simulink model "AME556_Project_Task3_v5"  (R2024b)
settings: Solver=daessc  StartTime=0.0  StopTime=10  FixedStep=0.0005  MaxStep=1e-3  RelTol=1e-2
InitFcn:
  | global params;
  | 
  | % Mass and geometry
  | params.m = 0.25;
  | params.l = 0.22;
  | params.mb = 8;
  | params.a = 0.25;
  | params.b = 0.15;
  | params.g = [0; 9.81; 0];
  | 
  | % Moment of inerita
  | Il_zz = params.m * params.l^2 / 12;
  | Ib_xx = params.mb * params.a^2 / 12;
  | Ib_yy = params.mb * params.b^2 / 12;
  | Ib_zz = params.mb * (params.a^2 + params.b^2) / 12;
  | params.Ib = diag([Ib_xx Ib_yy Ib_zz]);
  | 
  | % Spatial contact force parameters
  | Kp_g = 1e5;
  | Kd_g = 1e3;
  | 
  | % Ground contact positions
  | params.P1 = [0.0197; 0.0022; 0];
  | params.P2 = [0.1838; 0.0041; 0];
  | 
  | % State variables
  | q0 = [0.1; 0.45; 0; -pi/3; pi/2; -pi/6; pi/2]; % Initial states (before landing)
  | params.p_d = [0; 0.5; 0]; % Desired positions (after standing): [x_d; y_d; z_d];
  | params.theta_d = 0; % Desired angle
values from neighbouring files (symbols this model uses):
  dt = 0.04    [AME556_Project_Task3_Setup.m]
  N = 10    [AME556_Project_Task3_Setup.m]
undefined symbols (not defined in the file or in its folder): P1_world0, P2_world0, X, Y, Z
libraries: nesl_utility x27, sm_lib x23
settings Model: Creator=lewis  LastModifiedBy=zhaoshuai
settings SolverCC: DaesscMode=Balanced  AlgebraicLoopSolver=TrustRegion  MaxZcPerStep=1
settings DebuggingCC: UnconnectedInputMsg=warning  UnconnectedOutputMsg=warning  UnconnectedLineMsg=warning  SymbolicDimsDataTypeCodeGenerationDiagnostic=none
settings ModelReferenceCC: EnableRefExpFcnMdlSchedulingChecks=on
settings SFSimCC: CustomCodeUndefinedFunction=UseInterfaceOnly
settings RTWCC: GPUComputeCapability=3.5  DLArmComputeVersion=19.05
settings SimscapeCC: SimscapeLogType=all  SimscapeLogSimulationStatistics=on  SimscapeLogDataHistory=10000
settings ExplorerConfigSet: InternalSimMechanicsExplorerSettings="<ExplorerConfiguration><canonicalview>planar_xy</canonicalview><AnimationSetting><BasePlaybackSpeed>1.0</BasePlaybackSpeed><PlaybackSpeedFactor>1.0</PlaybackSpeedFactor></AnimationSetting><TilePanel><TileInfo><Tiles Columns=\"1\" Count=\"1\" Rows=\"1\"><Column Weight=\"1\"/><Row Weight=\"1\"/><Tile Height=\"1\" Width=\"1\" X=\"0\" Y=\"0\"/></Tiles></TileInfo><SceneInfo><SceneViewer><BGColor><R>0.60000002384185791</R><G>0.60000002384185791</G><B>0.60000002384185791</B></BGColor><Camera><DoPerspective>off</DoPerspective><Position><X>5.0000003994890756</X><Y>0.276248430591055971</Y><Z>5.31649358666460525</Z></Position><Center><X>5.0000003994890756</X><Y>0.276248430591055971</Y><Z>8.29291000314924531e-08</Z></Center><Up><X>0</X><Y>1</Y><Z>0</Z></Up><ViewLimDist>1</ViewLimDist><YLim>3.59969072164948445</YLim><XLim>5.40749999999999975</XLim></Camera></SceneViewer></SceneInfo></TilePanel><MechEditorPanel><Cameras/><GfxPanelCameraMap/><VideoCreator><PlaybackSpeedRatio>1.0</PlaybackSpeedRatio><FrameRate>60</FrameRate><VideoFormat>MPEG-4</VideoFormat><FrameSize>[1280 720]</FrameSize></VideoCreator></MechEditorPanel></ExplorerConfiguration>"

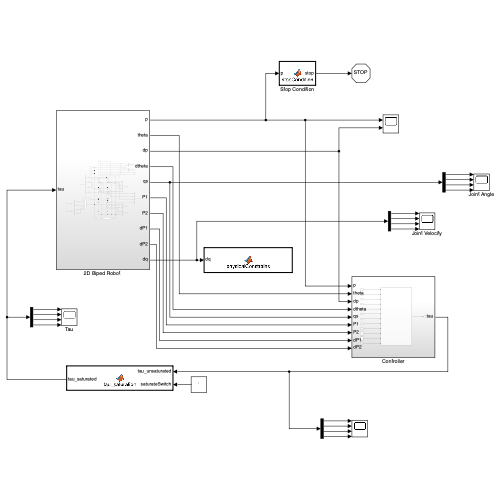
[thumbnail: Simulink's stored preview of the top-level diagram]
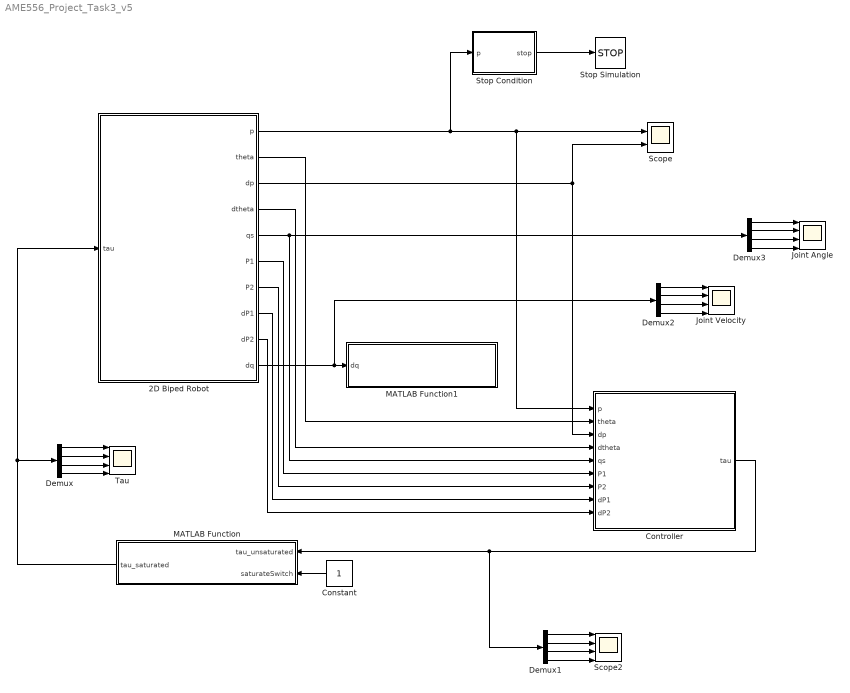
== system AME556_Project_Task3_v5 ==
  "2D Biped Robot " : Subsystem
  Constant : Constant
  Controller : Subsystem
  Demux{,1..3} (4 alike) : Demux
  Joint Angle : Scope  NumInputPorts=4
  Joint Velocity : Scope  NumInputPorts=4
  MATLAB Function : MATLAB Function  TreatAsAtomicUnit=on
  MATLAB Function1 : MATLAB Function  TreatAsAtomicUnit=on
  Scope : Scope  NumInputPorts=2
  Scope2 : Scope  NumInputPorts=4
  Stop Condition : MATLAB Function  TreatAsAtomicUnit=on
  Stop Simulation : Stop
  Tau : Scope  NumInputPorts=4
  wires:
  "2D Biped Robot "/1(p) -> Stop Condition/1(p), Scope/1, Controller/1(p)
  "2D Biped Robot "/2(theta) -> Controller/2(theta)
  "2D Biped Robot "/4(dtheta) -> Controller/4(dtheta)
  "2D Biped Robot "/6(P1) -> Controller/6(P1)
  "2D Biped Robot "/7(P2) -> Controller/7(P2)
  "2D Biped Robot "/8(dP1) -> Controller/8(dP1)
  "2D Biped Robot "/9(dP2) -> Controller/9(dP2)
  Stop Condition/1(stop) -> Stop Simulation/1
  "2D Biped Robot "/10(dq) -> Demux2/1, MATLAB Function1/1(dq)
  Constant/1 -> MATLAB Function/2(saturateSwitch)
  Demux/1 -> Tau/1
  Demux/2 -> Tau/2
  Demux/3 -> Tau/3
  Demux/4 -> Tau/4
  MATLAB Function/1(tau_saturated) -> Demux/1, "2D Biped Robot "/1(tau)
  Controller/1(tau) -> Demux1/1, MATLAB Function/1(tau_unsaturated)
  Demux1/1 -> Scope2/1
  Demux1/2 -> Scope2/2
  Demux1/3 -> Scope2/3
  Demux1/4 -> Scope2/4
  "2D Biped Robot "/3(dp) -> Scope/2, Controller/3(dp)
  Demux2/4 -> Joint Velocity/4
  Demux2/1 -> Joint Velocity/1
  Demux2/3 -> Joint Velocity/3
  Demux2/2 -> Joint Velocity/2
  Demux3/3 -> Joint Angle/3
  Demux3/1 -> Joint Angle/1
  Demux3/2 -> Joint Angle/2
  Demux3/4 -> Joint Angle/4
  "2D Biped Robot "/5(qs) -> Controller/5(qs), Demux3/1

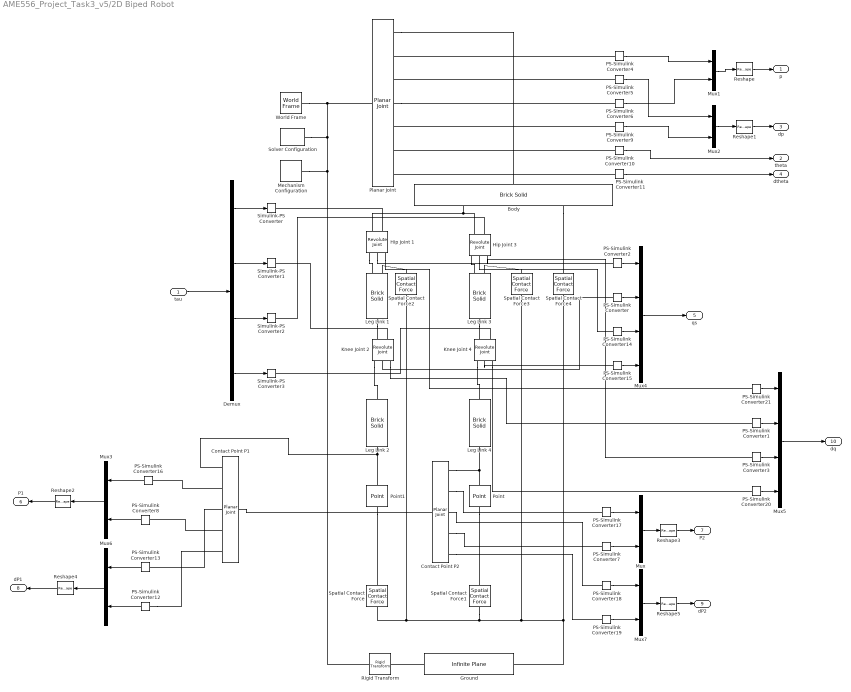
== system AME556_Project_Task3_v5/2D Biped Robot  ==
  tau : Inport
  Body : sm_lib/Body Elements/Brick Solid  BrickDimensions=[params.b params.a 0.1]  BrickDimensionsUnits=m  ExportEntireGeometry=on  InertiaType=Custom  BasedOnType=Density  Density=1000  DensityUnits=kg/m^3  Mass=params.mb  MassUnits=kg  CenterOfMass=[0 0 0]  CenterOfMassUnits=m  MomentsOfInertia=[0 0 Ib_zz]  MomentsOfInertiaUnits=kg*m^2  ProductsOfInertia=[0 0 0]  ProductsOfInertiaUnits=kg*m^2  GraphicType=FromGeometry  MarkerShape=Sphere  MarkerSize=10  GraphicVisPropType=SimpleVisualProperties  GraphicDiffuseColor=[0.5 0.5 0.5]  GraphicOpacity=1  GraphicSpecularColor=[0.5 0.5 0.5 1.0]  GraphicAmbientColor=[0.15 0.15 0.15 1.0]  GraphicEmissiveColor=[0.0 0.0 0.0 1.0]  GraphicShininess=75  DoExposeReferenceFrame=on  SerializedFrames=<Frames><Frame><Id>Frame1</Id><Value><Name>F</Name><Origin><Source>GeometricFeature</Source><FeatureName>-y surface</FeatureName></Origin><PrimaryAxis><DefinedDirection>+Z</DefinedDirection><Source>ReferenceFrame</Source><SourceDirection>+Z</SourceDirection><FeatureName></FeatureName></PrimaryAxis><SecondaryAxis><DefinedDirection>+X</DefinedDirection><Source>ReferenceFrame</Source><SourceDirection>+X</SourceDirection><FeatureName></FeatureName></SecondaryAxis></Value></Frame></Frames>
  Contact Point P1 : sm_lib/Joints/Planar Joint  JointMode=Normal  CompositeWrenchDir=FollowerOnBase  CompositeWrenchFrame=BaseFrame  SenseConstraintForce=off  SenseConstraintTorque=off  SenseTotalForce=off  SenseTotalTorque=off  PxPositionTargetSpecify=off  PxPositionTargetPriority=High  PxPositionTargetValue=P1_world0(1)  PxPositionTargetValueUnits=m  PxVelocityTargetSpecify=off  PxVelocityTargetPriority=High  PxVelocityTargetValue=0  PxVelocityTargetValueUnits=m/s  PxEquilibriumPosition=0  PxEquilibriumPositionUnits=m  PxSpringStiffness=0  PxSpringStiffnessUnits=N/m  PxDampingCoefficient=0  PxDampingCoefficientUnits=N/(m/s)  PxLowerLimitSpecify=off  PxLowerLimitBound=-1  PxLowerLimitBoundUnits=m  PxLowerLimitStiffness=1e6  PxLowerLimitStiffnessUnits=N/m  PxLowerLimitDamping=1e3  PxLowerLimitDampingUnits=N/(m/s)  PxLowerLimitTransitionRegionWidth=1e-4  PxLowerLimitTransitionRegionWidthUnits=m  PxUpperLimitSpecify=off  PxUpperLimitBound=1  PxUpperLimitBoundUnits=m  PxUpperLimitStiffness=1e6  PxUpperLimitStiffnessUnits=N/m  PxUpperLimitDamping=1e3  PxUpperLimitDampingUnits=N/(m/s)  PxUpperLimitTransitionRegionWidth=1e-4  PxUpperLimitTransitionRegionWidthUnits=m  PxTorqueActuationMode=NoTorque  PxMotionActuationMode=ComputedMotion  PxSensePosition=on  PxSenseVelocity=on  PxSenseAcceleration=off  PxSenseTorqueForce=off  PxSenseLowerLimitTorqueForce=off  PxSenseUpperLimitTorqueForce=off  PyPositionTargetSpecify=off  PyPositionTargetPriority=High  PyPositionTargetValue=P1_world0(2)  PyPositionTargetValueUnits=m  PyVelocityTargetSpecify=off  PyVelocityTargetPriority=High  PyVelocityTargetValue=0  PyVelocityTargetValueUnits=m/s  PyEquilibriumPosition=0  PyEquilibriumPositionUnits=m  PySpringStiffness=0  PySpringStiffnessUnits=N/m  PyDampingCoefficient=0  PyDampingCoefficientUnits=N/(m/s)  PyLowerLimitSpecify=off  PyLowerLimitBound=-1  PyLowerLimitBoundUnits=m  PyLowerLimitStiffness=1e6  PyLowerLimitStiffnessUnits=N/m  PyLowerLimitDamping=1e3  PyLowerLimitDampingUnits=N/(m/s)  PyLowerLimitTransitionRegionWidth=1e-4  PyLowerLimitTransitionRegionWidthUnits=m  PyUpperLimitSpecify=off  PyUpperLimitBound=1  PyUpperLimitBoundUnits=m  PyUpperLimitStiffness=1e6  PyUpperLimitStiffnessUnits=N/m  PyUpperLimitDamping=1e3  PyUpperLimitDampingUnits=N/(m/s)  PyUpperLimitTransitionRegionWidth=1e-4  PyUpperLimitTransitionRegionWidthUnits=m  PyTorqueActuationMode=NoTorque  PyMotionActuationMode=ComputedMotion  PySensePosition=on  PySenseVelocity=on  PySenseAcceleration=off  PySenseTorqueForce=off  PySenseLowerLimitTorqueForce=off  PySenseUpperLimitTorqueForce=off  RzPositionTargetSpecify=off  RzPositionTargetPriority=High  RzPositionTargetValue=q0(3)  RzPositionTargetValueUnits=deg  RzVelocityTargetSpecify=off  RzVelocityTargetPriority=High  RzVelocityTargetValue=0  RzVelocityTargetValueUnits=deg/s  RzEquilibriumPosition=0  RzEquilibriumPositionUnits=deg  RzSpringStiffness=0  RzSpringStiffnessUnits=N*m/deg  RzDampingCoefficient=0  RzDampingCoefficientUnits=N*m/(deg/s)  RzLowerLimitSpecify=off  RzLowerLimitBound=-90  RzLowerLimitBoundUnits=deg  RzLowerLimitStiffness=1e4  RzLowerLimitStiffnessUnits=N*m/deg  RzLowerLimitDamping=10  RzLowerLimitDampingUnits=N*m/(deg/s)  RzLowerLimitTransitionRegionWidth=0.1  RzLowerLimitTransitionRegionWidthUnits=deg  RzUpperLimitSpecify=off  RzUpperLimitBound=90  RzUpperLimitBoundUnits=deg  RzUpperLimitStiffness=1e4  RzUpperLimitStiffnessUnits=N*m/deg  RzUpperLimitDamping=10  RzUpperLimitDampingUnits=N*m/(deg/s)  RzUpperLimitTransitionRegionWidth=0.1  RzUpperLimitTransitionRegionWidthUnits=deg  RzTorqueActuationMode=NoTorque  RzMotionActuationMode=ComputedMotion  RzSensePosition=off  RzSenseVelocity=off  RzSenseAcceleration=off  RzSenseTorqueForce=off  RzSenseLowerLimitTorqueForce=off  RzSenseUpperLimitTorqueForce=off
  Contact Point P2 : sm_lib/Joints/Planar Joint  JointMode=Normal  CompositeWrenchDir=FollowerOnBase  CompositeWrenchFrame=BaseFrame  SenseConstraintForce=off  SenseConstraintTorque=off  SenseTotalForce=off  SenseTotalTorque=off  PxPositionTargetSpecify=off  PxPositionTargetPriority=High  PxPositionTargetValue=P2_world0(1)  PxPositionTargetValueUnits=m  PxVelocityTargetSpecify=off  PxVelocityTargetPriority=High  PxVelocityTargetValue=0  PxVelocityTargetValueUnits=m/s  PxEquilibriumPosition=0  PxEquilibriumPositionUnits=m  PxSpringStiffness=0  PxSpringStiffnessUnits=N/m  PxDampingCoefficient=0  PxDampingCoefficientUnits=N/(m/s)  PxLowerLimitSpecify=off  PxLowerLimitBound=-1  PxLowerLimitBoundUnits=m  PxLowerLimitStiffness=1e6  PxLowerLimitStiffnessUnits=N/m  PxLowerLimitDamping=1e3  PxLowerLimitDampingUnits=N/(m/s)  PxLowerLimitTransitionRegionWidth=1e-4  PxLowerLimitTransitionRegionWidthUnits=m  PxUpperLimitSpecify=off  PxUpperLimitBound=1  PxUpperLimitBoundUnits=m  PxUpperLimitStiffness=1e6  PxUpperLimitStiffnessUnits=N/m  PxUpperLimitDamping=1e3  PxUpperLimitDampingUnits=N/(m/s)  PxUpperLimitTransitionRegionWidth=1e-4  PxUpperLimitTransitionRegionWidthUnits=m  PxTorqueActuationMode=NoTorque  PxMotionActuationMode=ComputedMotion  PxSensePosition=on  PxSenseVelocity=on  PxSenseAcceleration=off  PxSenseTorqueForce=off  PxSenseLowerLimitTorqueForce=off  PxSenseUpperLimitTorqueForce=off  PyPositionTargetSpecify=off  PyPositionTargetPriority=High  PyPositionTargetValue=P2_world0(2)  PyPositionTargetValueUnits=m  PyVelocityTargetSpecify=off  PyVelocityTargetPriority=High  PyVelocityTargetValue=0  PyVelocityTargetValueUnits=m/s  PyEquilibriumPosition=0  PyEquilibriumPositionUnits=m  PySpringStiffness=0  PySpringStiffnessUnits=N/m  PyDampingCoefficient=0  PyDampingCoefficientUnits=N/(m/s)  PyLowerLimitSpecify=off  PyLowerLimitBound=-1  PyLowerLimitBoundUnits=m  PyLowerLimitStiffness=1e6  PyLowerLimitStiffnessUnits=N/m  PyLowerLimitDamping=1e3  PyLowerLimitDampingUnits=N/(m/s)  PyLowerLimitTransitionRegionWidth=1e-4  PyLowerLimitTransitionRegionWidthUnits=m  PyUpperLimitSpecify=off  PyUpperLimitBound=1  PyUpperLimitBoundUnits=m  PyUpperLimitStiffness=1e6  PyUpperLimitStiffnessUnits=N/m  PyUpperLimitDamping=1e3  PyUpperLimitDampingUnits=N/(m/s)  PyUpperLimitTransitionRegionWidth=1e-4  PyUpperLimitTransitionRegionWidthUnits=m  PyTorqueActuationMode=NoTorque  PyMotionActuationMode=ComputedMotion  PySensePosition=on  PySenseVelocity=on  PySenseAcceleration=off  PySenseTorqueForce=off  PySenseLowerLimitTorqueForce=off  PySenseUpperLimitTorqueForce=off  RzPositionTargetSpecify=off  RzPositionTargetPriority=High  RzPositionTargetValue=q0(3)  RzPositionTargetValueUnits=deg  RzVelocityTargetSpecify=off  RzVelocityTargetPriority=High  RzVelocityTargetValue=0  RzVelocityTargetValueUnits=deg/s  RzEquilibriumPosition=0  RzEquilibriumPositionUnits=deg  RzSpringStiffness=0  RzSpringStiffnessUnits=N*m/deg  RzDampingCoefficient=0  RzDampingCoefficientUnits=N*m/(deg/s)  RzLowerLimitSpecify=off  RzLowerLimitBound=-90  RzLowerLimitBoundUnits=deg  RzLowerLimitStiffness=1e4  RzLowerLimitStiffnessUnits=N*m/deg  RzLowerLimitDamping=10  RzLowerLimitDampingUnits=N*m/(deg/s)  RzLowerLimitTransitionRegionWidth=0.1  RzLowerLimitTransitionRegionWidthUnits=deg  RzUpperLimitSpecify=off  RzUpperLimitBound=90  RzUpperLimitBoundUnits=deg  RzUpperLimitStiffness=1e4  RzUpperLimitStiffnessUnits=N*m/deg  RzUpperLimitDamping=10  RzUpperLimitDampingUnits=N*m/(deg/s)  RzUpperLimitTransitionRegionWidth=0.1  RzUpperLimitTransitionRegionWidthUnits=deg  RzTorqueActuationMode=NoTorque  RzMotionActuationMode=ComputedMotion  RzSensePosition=off  RzSenseVelocity=off  RzSenseAcceleration=off  RzSenseTorqueForce=off  RzSenseLowerLimitTorqueForce=off  RzSenseUpperLimitTorqueForce=off
  Demux : Demux
  Ground : sm_lib/Curves and Surfaces/Infinite Plane  GraphicType=Rectangle  GraphicPlaneWidth=1  GraphicPlaneWidthUnits=m  GraphicPlaneHeight=10.5  GraphicPlaneHeightUnits=m  GraphicVisPropType=SimpleVisualProperties  GraphicDiffuseColor=[1 1 1]  GraphicOpacity=1  GraphicSpecularColor=[0.5 0.5 0.5 1.0]  GraphicAmbientColor=[0.15 0.15 0.15 1.0]  GraphicEmissiveColor=[0.0 0.0 0.0 1.0]  GraphicShininess=75
  Hip Joint 1 : sm_lib/Joints/Revolute Joint  JointMode=Normal  CompositeWrenchDir=FollowerOnBase  CompositeWrenchFrame=BaseFrame  SenseConstraintForce=off  SenseConstraintTorque=off  SenseTotalForce=off  SenseTotalTorque=off  PositionTargetSpecify=on  PositionTargetPriority=High  PositionTargetValue=params.q0(4)  PositionTargetValueUnits=rad  VelocityTargetSpecify=off  VelocityTargetPriority=High  VelocityTargetValue=0  VelocityTargetValueUnits=rad/s  EquilibriumPosition=0  EquilibriumPositionUnits=deg  SpringStiffness=0  SpringStiffnessUnits=N*m/deg  DampingCoefficient=0  DampingCoefficientUnits=N*m/(deg/s)  LowerLimitSpecify=on  LowerLimitBound=-120  LowerLimitBoundUnits=deg  LowerLimitStiffness=1e4  LowerLimitStiffnessUnits=N*m/deg  LowerLimitDamping=10  LowerLimitDampingUnits=N*m/(deg/s)  LowerLimitTransitionRegionWidth=0.1  LowerLimitTransitionRegionWidthUnits=deg  UpperLimitSpecify=on  UpperLimitBound=30  UpperLimitBoundUnits=deg  UpperLimitStiffness=1e4  UpperLimitStiffnessUnits=N*m/deg  UpperLimitDamping=10  UpperLimitDampingUnits=N*m/(deg/s)  UpperLimitTransitionRegionWidth=0.1  UpperLimitTransitionRegionWidthUnits=deg  TorqueActuationMode=InputTorque  MotionActuationMode=ComputedMotion  SensePosition=on  SenseVelocity=on  SenseAcceleration=off  SenseTorqueForce=off  SenseLowerLimitTorqueForce=off  SenseUpperLimitTorqueForce=off
  Hip Joint 3 : sm_lib/Joints/Revolute Joint  JointMode=Normal  CompositeWrenchDir=FollowerOnBase  CompositeWrenchFrame=BaseFrame  SenseConstraintForce=off  SenseConstraintTorque=off  SenseTotalForce=off  SenseTotalTorque=off  PositionTargetSpecify=on  PositionTargetPriority=High  PositionTargetValue=params.q0(6)  PositionTargetValueUnits=rad  VelocityTargetSpecify=off  VelocityTargetPriority=High  VelocityTargetValue=0  VelocityTargetValueUnits=rad/s  EquilibriumPosition=0  EquilibriumPositionUnits=deg  SpringStiffness=0  SpringStiffnessUnits=N*m/deg  DampingCoefficient=0  DampingCoefficientUnits=N*m/(deg/s)  LowerLimitSpecify=on  LowerLimitBound=-120  LowerLimitBoundUnits=deg  LowerLimitStiffness=1e4  LowerLimitStiffnessUnits=N*m/deg  LowerLimitDamping=10  LowerLimitDampingUnits=N*m/(deg/s)  LowerLimitTransitionRegionWidth=0.1  LowerLimitTransitionRegionWidthUnits=deg  UpperLimitSpecify=on  UpperLimitBound=30  UpperLimitBoundUnits=deg  UpperLimitStiffness=1e4  UpperLimitStiffnessUnits=N*m/deg  UpperLimitDamping=10  UpperLimitDampingUnits=N*m/(deg/s)  UpperLimitTransitionRegionWidth=0.1  UpperLimitTransitionRegionWidthUnits=deg  TorqueActuationMode=InputTorque  MotionActuationMode=ComputedMotion  SensePosition=on  SenseVelocity=on  SenseAcceleration=off  SenseTorqueForce=off  SenseLowerLimitTorqueForce=off  SenseUpperLimitTorqueForce=off
  Knee Joint 2 : sm_lib/Joints/Revolute Joint  JointMode=Normal  CompositeWrenchDir=FollowerOnBase  CompositeWrenchFrame=BaseFrame  SenseConstraintForce=off  SenseConstraintTorque=off  SenseTotalForce=off  SenseTotalTorque=off  PositionTargetSpecify=on  PositionTargetPriority=High  PositionTargetValue=params.q0(5)  PositionTargetValueUnits=rad  VelocityTargetSpecify=on  VelocityTargetPriority=High  VelocityTargetValue=0  VelocityTargetValueUnits=rad/s  EquilibriumPosition=0  EquilibriumPositionUnits=deg  SpringStiffness=0  SpringStiffnessUnits=N*m/deg  DampingCoefficient=0.035  DampingCoefficientUnits=N*m/(deg/s)  LowerLimitSpecify=on  LowerLimitBound=0  LowerLimitBoundUnits=deg  LowerLimitStiffness=1e4  LowerLimitStiffnessUnits=N*m/deg  LowerLimitDamping=10  LowerLimitDampingUnits=N*m/(deg/s)  LowerLimitTransitionRegionWidth=0.1  LowerLimitTransitionRegionWidthUnits=deg  UpperLimitSpecify=on  UpperLimitBound=160  UpperLimitBoundUnits=deg  UpperLimitStiffness=1e4  UpperLimitStiffnessUnits=N*m/deg  UpperLimitDamping=10  UpperLimitDampingUnits=N*m/(deg/s)  UpperLimitTransitionRegionWidth=0.1  UpperLimitTransitionRegionWidthUnits=deg  TorqueActuationMode=InputTorque  MotionActuationMode=ComputedMotion  SensePosition=on  SenseVelocity=on  SenseAcceleration=off  SenseTorqueForce=off  SenseLowerLimitTorqueForce=off  SenseUpperLimitTorqueForce=off
  Knee Joint 4 : sm_lib/Joints/Revolute Joint  JointMode=Normal  CompositeWrenchDir=FollowerOnBase  CompositeWrenchFrame=BaseFrame  SenseConstraintForce=off  SenseConstraintTorque=off  SenseTotalForce=off  SenseTotalTorque=off  PositionTargetSpecify=on  PositionTargetPriority=High  PositionTargetValue=params.q0(7)  PositionTargetValueUnits=rad  VelocityTargetSpecify=on  VelocityTargetPriority=High  VelocityTargetValue=0  VelocityTargetValueUnits=rad/s  EquilibriumPosition=0  EquilibriumPositionUnits=deg  SpringStiffness=0  SpringStiffnessUnits=N*m/deg  DampingCoefficient=0.035  DampingCoefficientUnits=N*m/(deg/s)  LowerLimitSpecify=on  LowerLimitBound=0  LowerLimitBoundUnits=deg  LowerLimitStiffness=1e4  LowerLimitStiffnessUnits=N*m/deg  LowerLimitDamping=10  LowerLimitDampingUnits=N*m/(deg/s)  LowerLimitTransitionRegionWidth=0.1  LowerLimitTransitionRegionWidthUnits=deg  UpperLimitSpecify=on  UpperLimitBound=160  UpperLimitBoundUnits=deg  UpperLimitStiffness=1e4  UpperLimitStiffnessUnits=N*m/deg  UpperLimitDamping=10  UpperLimitDampingUnits=N*m/(deg/s)  UpperLimitTransitionRegionWidth=0.1  UpperLimitTransitionRegionWidthUnits=deg  TorqueActuationMode=InputTorque  MotionActuationMode=ComputedMotion  SensePosition=on  SenseVelocity=on  SenseAcceleration=off  SenseTorqueForce=off  SenseLowerLimitTorqueForce=off  SenseUpperLimitTorqueForce=off
  Leg Link 1 : sm_lib/Body Elements/Brick Solid  BrickDimensions=[0.01 params.l 0.01]  BrickDimensionsUnits=m  ExportEntireGeometry=on  InertiaType=Custom  BasedOnType=Density  Density=1000  DensityUnits=kg/m^3  Mass=params.m  MassUnits=kg  CenterOfMass=[0 0 0]  CenterOfMassUnits=m  MomentsOfInertia=[0 0 Il_zz]  MomentsOfInertiaUnits=kg*m^2  ProductsOfInertia=[0 0 0]  ProductsOfInertiaUnits=kg*m^2  GraphicType=FromGeometry  MarkerShape=Sphere  MarkerSize=10  GraphicVisPropType=SimpleVisualProperties  GraphicDiffuseColor=[0.07451 0.6235 1]  GraphicOpacity=1  GraphicSpecularColor=[0.5 0.5 0.5 1.0]  GraphicAmbientColor=[0.15 0.15 0.15 1.0]  GraphicEmissiveColor=[0.0 0.0 0.0 1.0]  GraphicShininess=75  DoExposeReferenceFrame=off  SerializedFrames=<Frames><Frame><Id>Frame1</Id><Value><Name>top</Name><Origin><Source>GeometricFeature</Source><FeatureName>+y surface</FeatureName></Origin><PrimaryAxis><DefinedDirection>+Z</DefinedDirection><Source>ReferenceFrame</Source><SourceDirection>+Z</SourceDirection><FeatureName></FeatureName></PrimaryAxis><SecondaryAxis><DefinedDirection>+X</DefinedDirection><Source>ReferenceFrame</Source><SourceDirection>+X</SourceDirection><FeatureName></FeatureName></SecondaryAxis></Value></Frame><Frame><Id>Frame2</Id><Value><Name>bottom</Name><Origin><Source>GeometricFeature</Source><FeatureName>-y surface</FeatureName></Origin><PrimaryAxis><DefinedDirection>+Z</DefinedDirection><Source>ReferenceFrame</Source><SourceDirection>+Z</SourceDirection><FeatureName></FeatureName></PrimaryAxis><SecondaryAxis><DefinedDirection>+X</DefinedDirection><Source>ReferenceFrame</Source><SourceDirection>+X</SourceDirection><FeatureName></FeatureName></SecondaryAxis></Value></Frame></Frames>
  Leg Link 2 : sm_lib/Body Elements/Brick Solid  BrickDimensions=[0.01 params.l 0.01]  BrickDimensionsUnits=m  ExportEntireGeometry=off  InertiaType=Custom  BasedOnType=Density  Density=1000  DensityUnits=kg/m^3  Mass=params.m  MassUnits=kg  CenterOfMass=[0 0 0]  CenterOfMassUnits=m  MomentsOfInertia=[0 0 Il_zz]  MomentsOfInertiaUnits=kg*m^2  ProductsOfInertia=[0 0 0]  ProductsOfInertiaUnits=kg*m^2  GraphicType=FromGeometry  MarkerShape=Sphere  MarkerSize=10  GraphicVisPropType=SimpleVisualProperties  GraphicDiffuseColor=[1 0 0]  GraphicOpacity=1  GraphicSpecularColor=[0.5 0.5 0.5 1.0]  GraphicAmbientColor=[0.15 0.15 0.15 1.0]  GraphicEmissiveColor=[0.0 0.0 0.0 1.0]  GraphicShininess=75  DoExposeReferenceFrame=off  SerializedFrames=<Frames><Frame><Id>Frame1</Id><Value><Name>top</Name><Origin><Source>GeometricFeature</Source><FeatureName>+y surface</FeatureName></Origin><PrimaryAxis><DefinedDirection>+Z</DefinedDirection><Source>ReferenceFrame</Source><SourceDirection>+Z</SourceDirection><FeatureName></FeatureName></PrimaryAxis><SecondaryAxis><DefinedDirection>+X</DefinedDirection><Source>ReferenceFrame</Source><SourceDirection>+X</SourceDirection><FeatureName></FeatureName></SecondaryAxis></Value></Frame><Frame><Id>Frame2</Id><Value><Name>bottom</Name><Origin><Source>GeometricFeature</Source><FeatureName>-y surface</FeatureName></Origin><PrimaryAxis><DefinedDirection>+Z</DefinedDirection><Source>ReferenceFrame</Source><SourceDirection>+Z</SourceDirection><FeatureName></FeatureName></PrimaryAxis><SecondaryAxis><DefinedDirection>+X</DefinedDirection><Source>ReferenceFrame</Source><SourceDirection>+X</SourceDirection><FeatureName></FeatureName></SecondaryAxis></Value></Frame></Frames>
  Leg Link 3 : sm_lib/Body Elements/Brick Solid  BrickDimensions=[0.01 params.l 0.01]  BrickDimensionsUnits=m  ExportEntireGeometry=on  InertiaType=Custom  BasedOnType=Density  Density=1000  DensityUnits=kg/m^3  Mass=params.m  MassUnits=kg  CenterOfMass=[0 0 0]  CenterOfMassUnits=m  MomentsOfInertia=[0 0 Il_zz]  MomentsOfInertiaUnits=kg*m^2  ProductsOfInertia=[0 0 0]  ProductsOfInertiaUnits=kg*m^2  GraphicType=FromGeometry  MarkerShape=Sphere  MarkerSize=10  GraphicVisPropType=SimpleVisualProperties  GraphicDiffuseColor=[0 1 0]  GraphicOpacity=1  GraphicSpecularColor=[0.5 0.5 0.5 1.0]  GraphicAmbientColor=[0.15 0.15 0.15 1.0]  GraphicEmissiveColor=[0.0 0.0 0.0 1.0]  GraphicShininess=75  DoExposeReferenceFrame=off  SerializedFrames=<Frames><Frame><Id>Frame1</Id><Value><Name>top</Name><Origin><Source>GeometricFeature</Source><FeatureName>+y surface</FeatureName></Origin><PrimaryAxis><DefinedDirection>+Z</DefinedDirection><Source>ReferenceFrame</Source><SourceDirection>+Z</SourceDirection><FeatureName></FeatureName></PrimaryAxis><SecondaryAxis><DefinedDirection>+X</DefinedDirection><Source>ReferenceFrame</Source><SourceDirection>+X</SourceDirection><FeatureName></FeatureName></SecondaryAxis></Value></Frame><Frame><Id>Frame2</Id><Value><Name>bottom</Name><Origin><Source>GeometricFeature</Source><FeatureName>-y surface</FeatureName></Origin><PrimaryAxis><DefinedDirection>+Z</DefinedDirection><Source>ReferenceFrame</Source><SourceDirection>+Z</SourceDirection><FeatureName></FeatureName></PrimaryAxis><SecondaryAxis><DefinedDirection>+X</DefinedDirection><Source>ReferenceFrame</Source><SourceDirection>+X</SourceDirection><FeatureName></FeatureName></SecondaryAxis></Value></Frame></Frames>
  Leg Link 4 : sm_lib/Body Elements/Brick Solid  BrickDimensions=[0.01 params.l 0.01]  BrickDimensionsUnits=m  ExportEntireGeometry=off  InertiaType=Custom  BasedOnType=Density  Density=1000  DensityUnits=kg/m^3  Mass=params.m  MassUnits=kg  CenterOfMass=[0 0 0]  CenterOfMassUnits=m  MomentsOfInertia=[0 0 Il_zz]  MomentsOfInertiaUnits=kg*m^2  ProductsOfInertia=[0 0 0]  ProductsOfInertiaUnits=kg*m^2  GraphicType=FromGeometry  MarkerShape=Sphere  MarkerSize=10  GraphicVisPropType=SimpleVisualProperties  GraphicDiffuseColor=[1 1 0]  GraphicOpacity=1  GraphicSpecularColor=[0.5 0.5 0.5 1.0]  GraphicAmbientColor=[0.15 0.15 0.15 1.0]  GraphicEmissiveColor=[0.0 0.0 0.0 1.0]  GraphicShininess=75  DoExposeReferenceFrame=off  SerializedFrames=<Frames><Frame><Id>Frame1</Id><Value><Name>top</Name><Origin><Source>GeometricFeature</Source><FeatureName>+y surface</FeatureName></Origin><PrimaryAxis><DefinedDirection>+Z</DefinedDirection><Source>ReferenceFrame</Source><SourceDirection>+Z</SourceDirection><FeatureName></FeatureName></PrimaryAxis><SecondaryAxis><DefinedDirection>+X</DefinedDirection><Source>ReferenceFrame</Source><SourceDirection>+X</SourceDirection><FeatureName></FeatureName></SecondaryAxis></Value></Frame><Frame><Id>Frame2</Id><Value><Name>bottom</Name><Origin><Source>GeometricFeature</Source><FeatureName>-y surface</FeatureName></Origin><PrimaryAxis><DefinedDirection>+Z</DefinedDirection><Source>ReferenceFrame</Source><SourceDirection>+Z</SourceDirection><FeatureName></FeatureName></PrimaryAxis><SecondaryAxis><DefinedDirection>+X</DefinedDirection><Source>ReferenceFrame</Source><SourceDirection>+X</SourceDirection><FeatureName></FeatureName></SecondaryAxis></Value></Frame></Frames>
  Mechanism Configuration : sm_lib/Utilities/Mechanism Configuration  UniformGravity=Constant  GravityVector=-params.g  GravityVectorUnits=m/s^2  LinearizationDelta=0.001  JointModeTransitionNonlinearIterations=2
  Mux{,1..3,6..7} (6 alike) : Mux  Inputs=2
  Mux4 : Mux
  Mux5 : Mux
  PS-Simulink Converter{,1..21} (22 alike) : nesl_utility/PS-Simulink Converter  PhysicalDomain=network_engine_domain  SubClassName=ps_output  LeftPortType=input  RightPortType=output  PseudoPeriodic=off  Frequencies=[]  VectorFormat=inherit  Unit=inherit  AffineConversion=off
  Planar Joint : sm_lib/Joints/Planar Joint  JointMode=Normal  CompositeWrenchDir=FollowerOnBase  CompositeWrenchFrame=BaseFrame  SenseConstraintForce=off  SenseConstraintTorque=off  SenseTotalForce=off  SenseTotalTorque=off  PxPositionTargetSpecify=on  PxPositionTargetPriority=High  PxPositionTargetValue=params.q0(1)  PxPositionTargetValueUnits=m  PxVelocityTargetSpecify=off  PxVelocityTargetPriority=High  PxVelocityTargetValue=0  PxVelocityTargetValueUnits=m/s  PxEquilibriumPosition=0  PxEquilibriumPositionUnits=m  PxSpringStiffness=0  PxSpringStiffnessUnits=N/m  PxDampingCoefficient=0  PxDampingCoefficientUnits=N/(m/s)  PxLowerLimitSpecify=off  PxLowerLimitBound=-1  PxLowerLimitBoundUnits=m  PxLowerLimitStiffness=1e6  PxLowerLimitStiffnessUnits=N/m  PxLowerLimitDamping=1e3  PxLowerLimitDampingUnits=N/(m/s)  PxLowerLimitTransitionRegionWidth=1e-4  PxLowerLimitTransitionRegionWidthUnits=m  PxUpperLimitSpecify=off  PxUpperLimitBound=1  PxUpperLimitBoundUnits=m  PxUpperLimitStiffness=1e6  PxUpperLimitStiffnessUnits=N/m  PxUpperLimitDamping=1e3  PxUpperLimitDampingUnits=N/(m/s)  PxUpperLimitTransitionRegionWidth=1e-4  PxUpperLimitTransitionRegionWidthUnits=m  PxTorqueActuationMode=NoTorque  PxMotionActuationMode=ComputedMotion  PxSensePosition=on  PxSenseVelocity=on  PxSenseAcceleration=off  PxSenseTorqueForce=off  PxSenseLowerLimitTorqueForce=off  PxSenseUpperLimitTorqueForce=off  PyPositionTargetSpecify=on  PyPositionTargetPriority=High  PyPositionTargetValue=params.q0(2)  PyPositionTargetValueUnits=m  PyVelocityTargetSpecify=off  PyVelocityTargetPriority=High  PyVelocityTargetValue=0  PyVelocityTargetValueUnits=m/s  PyEquilibriumPosition=0  PyEquilibriumPositionUnits=m  PySpringStiffness=0  PySpringStiffnessUnits=N/m  PyDampingCoefficient=0  PyDampingCoefficientUnits=N/(m/s)  PyLowerLimitSpecify=off  PyLowerLimitBound=-1  PyLowerLimitBoundUnits=m  PyLowerLimitStiffness=1e6  PyLowerLimitStiffnessUnits=N/m  PyLowerLimitDamping=1e3  PyLowerLimitDampingUnits=N/(m/s)  PyLowerLimitTransitionRegionWidth=1e-4  PyLowerLimitTransitionRegionWidthUnits=m  PyUpperLimitSpecify=off  PyUpperLimitBound=1  PyUpperLimitBoundUnits=m  PyUpperLimitStiffness=1e6  PyUpperLimitStiffnessUnits=N/m  PyUpperLimitDamping=1e3  PyUpperLimitDampingUnits=N/(m/s)  PyUpperLimitTransitionRegionWidth=1e-4  PyUpperLimitTransitionRegionWidthUnits=m  PyTorqueActuationMode=NoTorque  PyMotionActuationMode=ComputedMotion  PySensePosition=on  PySenseVelocity=on  PySenseAcceleration=off  PySenseTorqueForce=off  PySenseLowerLimitTorqueForce=off  PySenseUpperLimitTorqueForce=off  RzPositionTargetSpecify=on  RzPositionTargetPriority=High  RzPositionTargetValue=params.q0(3)  RzPositionTargetValueUnits=rad  RzVelocityTargetSpecify=off  RzVelocityTargetPriority=High  RzVelocityTargetValue=0  RzVelocityTargetValueUnits=deg/s  RzEquilibriumPosition=0  RzEquilibriumPositionUnits=deg  RzSpringStiffness=0  RzSpringStiffnessUnits=N*m/deg  RzDampingCoefficient=0  RzDampingCoefficientUnits=N*m/(deg/s)  RzLowerLimitSpecify=off  RzLowerLimitBound=-90  RzLowerLimitBoundUnits=deg  RzLowerLimitStiffness=1e4  RzLowerLimitStiffnessUnits=N*m/deg  RzLowerLimitDamping=10  RzLowerLimitDampingUnits=N*m/(deg/s)  RzLowerLimitTransitionRegionWidth=0.1  RzLowerLimitTransitionRegionWidthUnits=deg  RzUpperLimitSpecify=off  RzUpperLimitBound=90  RzUpperLimitBoundUnits=deg  RzUpperLimitStiffness=1e4  RzUpperLimitStiffnessUnits=N*m/deg  RzUpperLimitDamping=10  RzUpperLimitDampingUnits=N*m/(deg/s)  RzUpperLimitTransitionRegionWidth=0.1  RzUpperLimitTransitionRegionWidthUnits=deg  RzTorqueActuationMode=NoTorque  RzMotionActuationMode=ComputedMotion  RzSensePosition=on  RzSenseVelocity=on  RzSenseAcceleration=off  RzSenseTorqueForce=off  RzSenseLowerLimitTorqueForce=off  RzSenseUpperLimitTorqueForce=off
  Point : sm_lib/Curves and Surfaces/Point  GraphicType=Marker  MarkerShape=Sphere  MarkerSize=10  GraphicVisPropType=SimpleVisualProperties  GraphicDiffuseColor=[1 1 0.06667]  GraphicOpacity=1  GraphicSpecularColor=[0.5 0.5 0.5 1.0]  GraphicAmbientColor=[0.15 0.15 0.15 1.0]  GraphicEmissiveColor=[0.0 0.0 0.0 1.0]  GraphicShininess=75
  Point1 : sm_lib/Curves and Surfaces/Point  GraphicType=Marker  MarkerShape=Sphere  MarkerSize=10  GraphicVisPropType=SimpleVisualProperties  GraphicDiffuseColor=[1 0 0]  GraphicOpacity=1  GraphicSpecularColor=[0.5 0.5 0.5 1.0]  GraphicAmbientColor=[0.15 0.15 0.15 1.0]  GraphicEmissiveColor=[0.0 0.0 0.0 1.0]  GraphicShininess=75
  Reshape{,1..5} (6 alike) : Reshape  OutputDimensionality=Customize  OutputDimensions=[2,1]
  Rigid Transform : sm_lib/Frames and Transforms/Rigid Transform  RotationMethod=AlignedAxes  FollAlignAxisA=+X  BaseAlignAxisA=+Z  FollAlignAxisB=+Y  BaseAlignAxisB=+X  RotationStandardAxis=+Z  RotationAngle=0  RotationAngleUnits=deg  RotationArbitraryAxis=[0 0 1]  RotationSequenceAxes=FollowerAxes  RotationSequence=XYX  RotationSequenceAngles=[0 0 0]  RotationSequenceAnglesUnits=deg  RotationMatrix=[1 0 0;0 1 0;0 0 1]  Quaternion=[1 0 0 0]  TranslationMethod=StandardAxis  TranslationCartesianOffset=[0 0 0]  TranslationCartesianOffsetUnits=m  TranslationStandardAxis=+X  TranslationStandardOffset=5  TranslationStandardOffsetUnits=m  TranslationROffset=0  TranslationROffsetUnits=m  TranslationThetaOffset=0  TranslationThetaOffsetUnits=deg  TranslationZOffset=0  TranslationZOffsetUnits=m
  Simulink-PS Converter{,1..3} (4 alike) : nesl_utility/Simulink-PS Converter  PhysicalDomain=network_engine_domain  SubClassName=ps_input  LeftPortType=input  RightPortType=output  PseudoPeriodic=off  Frequencies=[]  NoiseDistribution=none  NoiseParameters=[]  Unit=1  AffineConversion=off  FilteringAndDerivatives=provide  SimscapeFilterOrder=1  InputFilterTimeConstant=0.001  UdotUserProvided=0
  Solver Configuration : nesl_utility/Solver Configuration  PhysicalDomain=network_engine_domain  SubClassName=solver  LeftPortType=input  RightPortType=generic  Tones=[]  Harmonics=[]  SimulateNoise=off  Profile=off  UseLocalSampling=off  EnableSwitchedLinearOptims=on  FrequencyDomain=off  UseCCode=off  RelTol=0.001  AbsTol=1e-06  MinStep=1e-09  ToWorkspace=off  RevertToSquareIcSolve=off  NumHomotopyIterations=100  PhasorMode=off  PhasorModeNumHarmonics=1  ConsistencySolver=NEWTON_XTOL_AFTER_FTOL  IndexReductionMethod=DerivativeReplacement  DoDC=off  ResidualTolerance=1e-09  ConsistencyTolSource=GLOBAL  ConsistencyAbsTol=0.001  ConsistencyRelTol=0.001  ConsistencyTolFactor=0.001  UseLocalSolver=off  LocalSolverChoice=NE_BACKWARD_EULER_ADVANCER  ResolveIndetEquations=on  FunctionEvalNumThread=1  LocalSolverSampleTime=0.001  DoFixedCost=off  MaxNonlinIter=3  MaxModeIter=2  ComputeImpulses=off  ImpulseIterations=2  LinearAlgebra=auto  LinearAlgebraNumThread=0  EquationFormulation=NE_TIME_EF  DelaysMemoryBudget=1024  AutomaticFiltering=on  FilteringTimeConstant=0.001  PartitionStorageMethod=AS_NEEDED  PartitionMemoryBudget=1024  PartitionMethod=ROBUST  MultibodyUseLocalSolver=off  MultibodyLocalSolverChoice=ODE1  MultibodyLocalSolverSampleTime=0.001
  Spatial Contact Force{,1..4} (5 alike) : sm_lib/Forces and Torques/Spatial Contact Force  NormalForceType=SmoothSpringDamper  NormalStiffness=Kp_g  NormalStiffnessUnits=N/m  NormalDamping=Kd_g  NormalDampingUnits=N/(m/s)  NormalTransitionRegionWidth=1e-4  NormalTransitionRegionWidthUnits=m  FrictionType=SmoothStickSlip  CoefficientOfStaticFriction=Cof_s  CoefficientOfDynamicFriction=Cof_d  FrictionalCriticalVelocity=1e-3  FrictionalCriticalVelocityUnits=m/s  SenseContactSignal=off  SensePenetrationDepth=off  SenseSeparationDistance=off  SenseNormalForceMagnitude=off  SenseFrictionalForceMagnitude=off  SenseNormalVelocity=off  SenseTangentialVelocity=off  SenseContactBaseRotation=off  SenseContactBaseTranslation=off  SenseContactFollowerRotation=off  SenseContactFollowerTranslation=off  ZeroCrossDetectContactStartAndEnd=off
  World Frame : sm_lib/Frames and Transforms/World Frame
  p : Outport
  theta : Outport  Port=2
  dp : Outport  Port=3
  dtheta : Outport  Port=4
  qs : Outport  Port=5
  P1 : Outport  Port=6
  P2 : Outport  Port=7
  dP1 : Outport  Port=8
  dP2 : Outport  Port=9
  dq : Outport  Port=10
  wires:
  PS-Simulink Converter4/1 -> Mux1/1
  PS-Simulink Converter6/1 -> Mux1/2
  PS-Simulink Converter5/1 -> Mux2/1
  Demux/1 -> Simulink-PS Converter/1
  Demux/2 -> Simulink-PS Converter1/1
  Demux/3 -> Simulink-PS Converter2/1
  PS-Simulink Converter8/1 -> Mux3/2
  PS-Simulink Converter9/1 -> Mux2/2
  PS-Simulink Converter11/1 -> dtheta/1
  PS-Simulink Converter10/1 -> theta/1
  PS-Simulink Converter16/1 -> Mux3/1
  PS-Simulink Converter17/1 -> Mux/1
  PS-Simulink Converter7/1 -> Mux/2
  Mux/1 -> Reshape3/1
  Mux1/1 -> Reshape/1
  Mux2/1 -> Reshape1/1
  Mux3/1 -> Reshape2/1
  Reshape/1 -> p/1
  Reshape1/1 -> dp/1
  Reshape3/1 -> P2/1
  Reshape2/1 -> P1/1
  PS-Simulink Converter15/1 -> Mux4/4
  PS-Simulink Converter14/1 -> Mux4/3
  PS-Simulink Converter/1 -> Mux4/2
  PS-Simulink Converter2/1 -> Mux4/1
  Mux4/1 -> qs/1
  Demux/4 -> Simulink-PS Converter3/1
  tau/1 -> Demux/1
  Mux6/1 -> Reshape4/1
  Reshape4/1 -> dP1/1
  PS-Simulink Converter13/1 -> Mux6/1
  PS-Simulink Converter12/1 -> Mux6/2
  PS-Simulink Converter18/1 -> Mux7/1
  Mux7/1 -> Reshape5/1
  Reshape5/1 -> dP2/1
  PS-Simulink Converter19/1 -> Mux7/2
  Mux5/1 -> dq/1
  PS-Simulink Converter1/1 -> Mux5/2
  PS-Simulink Converter3/1 -> Mux5/3
  PS-Simulink Converter21/1 -> Mux5/1
  PS-Simulink Converter20/1 -> Mux5/4
  connections:
  Spatial Contact Force4/LConn1 -- Spatial Contact Force2/LConn1 -- Spatial Contact Force/LConn1 -- Spatial Contact Force1/LConn1 -- Spatial Contact Force3/LConn1 -- Ground/RConn1
  Hip Joint 1/LConn1 -- Hip Joint 3/LConn1 -- Body/LConn1
  Planar Joint/RConn1 -- Body/RConn1
  Hip Joint 1/RConn1 -- Leg Link 1/LConn1
  Hip Joint 3/RConn1 -- Leg Link 3/LConn1
  Leg Link 1/RConn1 -- Knee Joint 2/LConn1
  Knee Joint 2/RConn1 -- Leg Link 2/LConn1
  Knee Joint 4/RConn1 -- Leg Link 4/LConn1
  Leg Link 3/RConn1 -- Knee Joint 4/LConn1
  Leg Link 1/LConn2 -- Spatial Contact Force2/RConn1
  Leg Link 3/LConn2 -- Spatial Contact Force3/RConn1
  Body/LConn2 -- Spatial Contact Force4/RConn1
  PS-Simulink Converter/LConn1 -- Knee Joint 2/RConn2
  Hip Joint 1/RConn2 -- PS-Simulink Converter2/LConn1
  PS-Simulink Converter4/LConn1 -- Planar Joint/RConn2
  PS-Simulink Converter5/LConn1 -- Planar Joint/RConn3
  Planar Joint/RConn4 -- PS-Simulink Converter6/LConn1
  Point1/RConn1 -- Spatial Contact Force/RConn1
  Point/RConn1 -- Spatial Contact Force1/RConn1
  Contact Point P2/RConn1 -- Point/LConn1 -- Leg Link 4/RConn1
  Contact Point P1/RConn1 -- Point1/LConn1 -- Leg Link 2/RConn1
  PS-Simulink Converter9/LConn1 -- Planar Joint/RConn5
  PS-Simulink Converter10/LConn1 -- Planar Joint/RConn6
  PS-Simulink Converter11/LConn1 -- Planar Joint/RConn7
  Hip Joint 3/RConn2 -- PS-Simulink Converter14/LConn1
  Knee Joint 4/RConn2 -- PS-Simulink Converter15/LConn1
  Hip Joint 1/LConn2 -- Simulink-PS Converter/RConn1
  Knee Joint 2/LConn2 -- Simulink-PS Converter1/RConn1
  Hip Joint 3/LConn2 -- Simulink-PS Converter2/RConn1
  Knee Joint 4/LConn2 -- Simulink-PS Converter3/RConn1
  Contact Point P1/RConn2 -- PS-Simulink Converter16/LConn1
  Contact Point P2/RConn2 -- PS-Simulink Converter17/LConn1
  World Frame/RConn1 -- Solver Configuration/RConn1 -- Contact Point P1/LConn1 -- Rigid Transform/LConn1 -- Contact Point P2/LConn1 -- Mechanism Configuration/RConn1 -- Planar Joint/LConn1
  Ground/LConn1 -- Rigid Transform/RConn1
  Contact Point P1/RConn4 -- PS-Simulink Converter8/LConn1
  Contact Point P1/RConn3 -- PS-Simulink Converter13/LConn1
  PS-Simulink Converter12/LConn1 -- Contact Point P1/RConn5
  Contact Point P2/RConn4 -- PS-Simulink Converter7/LConn1
  Contact Point P2/RConn3 -- PS-Simulink Converter18/LConn1
  Contact Point P2/RConn5 -- PS-Simulink Converter19/LConn1
  Hip Joint 1/RConn3 -- PS-Simulink Converter21/LConn1
  Knee Joint 2/RConn3 -- PS-Simulink Converter1/LConn1
  Hip Joint 3/RConn3 -- PS-Simulink Converter3/LConn1
  Knee Joint 4/RConn3 -- PS-Simulink Converter20/LConn1

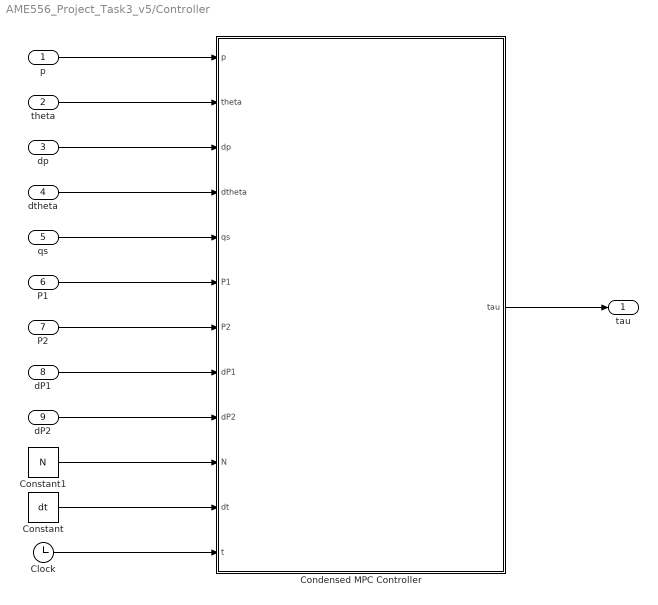
== system AME556_Project_Task3_v5/Controller ==
  p : Inport
  theta : Inport  Port=2
  dp : Inport  Port=3
  dtheta : Inport  Port=4
  qs : Inport  Port=5
  P1 : Inport  Port=6
  P2 : Inport  Port=7
  dP1 : Inport  Port=8
  dP2 : Inport  Port=9
  Clock : Clock
  Condensed MPC Controller : MATLAB Function  TreatAsAtomicUnit=on
  Constant : Constant  Value=dt
  Constant1 : Constant  Value=N
  tau : Outport
  wires:
  Condensed MPC Controller/1(tau) -> tau/1
  p/1 -> Condensed MPC Controller/1(p)
  theta/1 -> Condensed MPC Controller/2(theta)
  dp/1 -> Condensed MPC Controller/3(dp)
  P1/1 -> Condensed MPC Controller/6(P1)
  P2/1 -> Condensed MPC Controller/7(P2)
  dP1/1 -> Condensed MPC Controller/8(dP1)
  dP2/1 -> Condensed MPC Controller/9(dP2)
  Clock/1 -> Condensed MPC Controller/12(t)
  Constant1/1 -> Condensed MPC Controller/10(N)
  Constant/1 -> Condensed MPC Controller/11(dt)
  dtheta/1 -> Condensed MPC Controller/4(dtheta)
  qs/1 -> Condensed MPC Controller/5(qs)

== matlab function AME556_Project_Task3_v5/MATLAB Function ==
  data: tau_unsaturated input; tau_saturated output; saturateSwitch input
function tau_saturated = tau_saturation(tau_unsaturated, saturateSwitch)
    if saturateSwitch == 1
        tau_limits = [30, 60, 30, 60];
    
        tau_saturated = tau_unsaturated;
    
        for i = 1:length(tau_unsaturated)
            if tau_unsaturated(i) > tau_limits(i)
                tau_saturated(i) = tau_limits(i);
                warning('Tau %d (%.2f) is saturated to %d', i, tau_unsaturated(i), tau_limits(i));
            elseif tau_unsaturated(i) < -tau_limits(i)
                tau_saturated(i) = -tau_limits(i);
                warning('Tau %d (%.2f) is saturated to -%d', i, tau_unsaturated(i), tau_limits(i));
            end
        end
    else
        tau_saturated = tau_unsaturated;
    end
end

== matlab function AME556_Project_Task3_v5/Stop Condition ==
  data: p input; stop output
function stop = stopCondition(p)

x = p(1);

if x - 10 >= 0
    stop = 1;
else
    stop = 0;
end

end

== matlab function AME556_Project_Task3_v5/Controller/Condensed MPC Controller ==
  data: p input; theta input; dp input; dtheta input; qs input; tau output; P1 input; P2 input; dP1 input; dP2 input; N input; dt input; t input
%% Function: Low Level Control

function tau = lowLevelControl(p, theta, dp, dtheta, qs, P1, P2, dP1, dP2, N, dt, t)

    con = gaitSchedule(N, dt, t);
    F = condensed_mpc_controller(p, theta, dp, dtheta, P1, P2, N, dt, t, con);
    J = jacobianFcn(theta, qs);
    
    tau = zeros(4, 1);
    if con(1, 1) && con(2, 1)
        tau = -J' * F;
    elseif con(1, 1) && ~con(2, 1)
        F_swing = swingLegControl(p, dp, P2, dP2, N, dt, t);
        F_new = [F(1: 2); -F_swing];
        tau = -J' * F_new;
    elseif con(2, 1) && ~con(1, 1)
        F_swing = swingLegControl(p, dp, P1, dP1, N, dt, t);
        F_new = [-F_swing; F(3: 4)];
        tau = -J' * F_new;    
    else
        % 为了飞的修改：俩腿都swing
        F_swing1 = swingLegControl(p, dp, P1, dP1, N, dt, t);  
        F_swing2 = swingLegControl(p, dp, P2, dP2, N, dt, t); 
        F_new = [-F_swing1; -F_swing2];
        tau = -J' * F_new; 
        % 飞行修改结束
    end
end

%% Function: Condensed MPC Controller

function F = condensed_mpc_controller(p, theta, dp, dtheta, P1, P2, N, dt, t, con)

    % 为了飞的修改：~any(con(:, 1)) 任何一条腿都不为1（也就是都是0）的话，直接F=0
    if ~any(con(:, 1))
        F = zeros(4, 1); 
        return;
    end
    % 为了飞的修改结束

% Parameters
mt = 8;
a = 0.25;
b = 0.15;
g = [0; 9.81; 0];
Ib_zz = mt * (a^2 + b^2) / 12;

numStates = 7;
numCtrls = 4;
Q = diag([200 200 800 30 10 10 0]);
R = 0.0001*eye(numCtrls);

% q = [x; y; z; R1; dx; dy; dz; wbx; wby; wbz];
% X = [x; y; theta; dx; dy; dtheta; g];
X = zeros(numStates, 1);
X(1: 2) = p;
X(3) = theta;
X(4: 5) = dp;
X(6) = dtheta;
X(7) = g(2);

% Desired states
%acc = 0.3;
t1 = 1;
v1 = 0.5;
%v1 = acc * t1;
y_d = 0.4;
if t <= t1
    X_d = [1; y_d; 0; v1; 0; 0; g(2)];
else
    X_d = [v1*t; y_d; 0; v1; 0; 0; g(2)];
end

% Reference Trajectory
X_ref = getReferenceTrajectory(dt, N, p, theta, dp, dtheta, X_d);
y = reshape(X_ref, [numStates*N 1]);

r1 = P1 - p;
r2 = P2 - p;

% Linearized system (A, B)
A = [zeros(3)   eye(3)    zeros(3,1);
     zeros(3, numStates-1) [0; -1; 0];
     zeros(1, numStates)];

B = [zeros(3, numCtrls);
     eye(2)/mt eye(2)/mt;
     -r1(2)/Ib_zz r1(1)/Ib_zz -r2(2)/Ib_zz r2(1)/Ib_zz;
     zeros(1, numCtrls)];

% Discrete-time system matrices (Ak, Bk)
Ak = A * dt + eye(size(A, 1));
Bk = B * dt;

% Aqp
Aqp = [];
for i = 1: N
    Aqp = [Aqp; mpower(Ak, i)];
end

% bqp
Bqp = repmat(zeros(size(Bk)), N, N);
for i = 0: N-1
    element = mpower(Ak, i) * Bk;
    Bqp = Bqp + kron(diag(ones(1, N - i), -i), element);
end

% Condensation
L = kron(eye(N), Q);
K = kron(eye(N), R);

% Optimization weights (H, f)
H = 2*(Bqp'*L*Bqp + K);
f = 2*Bqp'*L*(Aqp*X - y);

% Inequality constraints (A_ineq, b_ineq)
Aineq_mu = kron(eye(2), [1 -0.7; -1 -0.7]);
Aineq_mu_N = kron(eye(N), Aineq_mu);
Aineq_F = kron(eye(2), [0 1; 0 -1]);
Aineq_F_N = kron(eye(N), Aineq_F);
Aineq = [Aineq_mu_N; Aineq_F_N];

bineq_mu = repmat([0; 0; 0; 0], N, 1);
bineq_f = [];
for i = 1: N
    bineq_f = [bineq_f; [250; -10]*con(1, i); [250; -10]*con(2, i)];
end
bineq = [bineq_mu; bineq_f];

% Initial guess
u0 = zeros(length(f), 1);

% Quadratic programming
options = optimoptions('quadprog', 'Algorithm', 'active-set', 'Display', 'off');
u_mpc = quadprog(H, f, Aineq, bineq, [], [], [], [], u0, options);

% Force inputs
F = u_mpc(1: numCtrls);

end

%% Function: Get Reference Geometry

function X_ref = getReferenceTrajectory(dt, N, p, theta, dp, dtheta, X_d)

X = [p; theta; dp; dtheta; 9.81];
X_ref = repmat(X, 1, N);

for i = 1: 3
    for k = 2: N
        if X_d(i + 3) ~= 0
            X_ref(i, k) = X(i) + X_d(i+3)*((k-1)*dt);
        else
            X_ref(i, k) = X_d(i);
        end
    end
end

end

%% Function: Swing Leg Control

function F_swing = swingLegControl(p, dp, P, dP, N, dt, t)

% Leg swing height
swingHeight = 0.1;

Kp = diag([200,300]);
Kd = eye(2)*5;

del_t = N*dt/2;
ts = rem(t, del_t);

% Desired leg positions
Px_d = p(1) + (1/2)*(del_t)*dp(1);
Py_d = swingHeight * sin(pi*ts/(del_t));

F_swing = Kp*([Px_d; Py_d] - P) + Kd*(0 - dP);

end

%% Function: Jacobian Function
% Convert contact forces to joint torques

function J = jacobianFcn(theta, qs)

l = 0.22;

q1 = qs(1); q2 = qs(2); q3 = qs(3); q4 = qs(4);

J = [l*cos(q1 + q2 + theta) + l*cos(q1 + theta), l*cos(q1 + q2 + theta),                                          0,                      0;
     l*sin(q1 + q2 + theta) + l*sin(q1 + theta), l*sin(q1 + q2 + theta),                                          0,                      0;
                                              0,                      0, l*cos(q3 + q4 + theta) + l*cos(q3 + theta), l*cos(q3 + q4 + theta);
                                              0,                      0, l*sin(q3 + q4 + theta) + l*sin(q3 + theta), l*sin(q3 + q4 + theta)];

end

%% Function: Gait Schedule
% Generate gait schedule based on walking phase

function sigma = gaitSchedule(N, dt, t)

phase = floor(t/dt);
k = rem(phase, N);

% 为了飞的修改：一部分双0
sigma_l0 = [1 1 1 1 0 0 0 0 0 0];
sigma_r0 = [0 0 0 0 0 1 1 1 1 0];
% 为了飞的修改结束

if k ~= 0
    sigma_l = [sigma_l0(k+1: N) sigma_l0(1: k)];
    sigma_r = [sigma_r0(k+1: N) sigma_r0(1: k)];
else
    sigma_l = sigma_l0;
    sigma_r = sigma_r0;
end

sigma = [sigma_l; sigma_r];

end

== matlab function AME556_Project_Task3_v5/MATLAB Function1 ==
  data: dq input
function physicalConstrains(dq) 
    % 定义每个关节的速度限制（单位：rad/s）
    jointVelocityLimits = [30, 15, 30, 15];
    
    % 将 dq 从 deg/s 转换为 rad/s
    dq_rad = dq; % 角度 -> 弧度转换

    % 遍历所有关节速度，检测是否超限
    for i = 1:length(dq_rad)
        if abs(dq_rad(i)) > jointVelocityLimits(i)
            warning('Joint %d velocity (%.2f rad/s) exceeds the limit! Limit: %.2f rad/s', ...
                    i, dq_rad(i), jointVelocityLimits(i));
        end
    end
end
